simulink model "wk10_clsys"  (R2022b)
settings: Solver=VariableStepAuto  StartTime=0.0  StopTime=75  RelTol=1e-3
model workspace (MAT data in the model file):
  seed = 0
values from neighbouring files (symbols this model uses):
  Kd = 3    [wk10_clsys_script.m]
  Ki = 6    [wk10_clsys_script.m]
  Kp = 0.35    [wk10_clsys_script.m]
  s_eed = floor(rand(1)*100)    [wk10_clsys_script.m]
  sd_noise = 0.1    [wk10_clsys_script.m]
  tau_f = 70    [wk10_clsys_script.m]
settings Model: Creator=sd87  LastModifiedBy=agjri
settings ModelReferenceCC: EnableRefExpFcnMdlSchedulingChecks=on

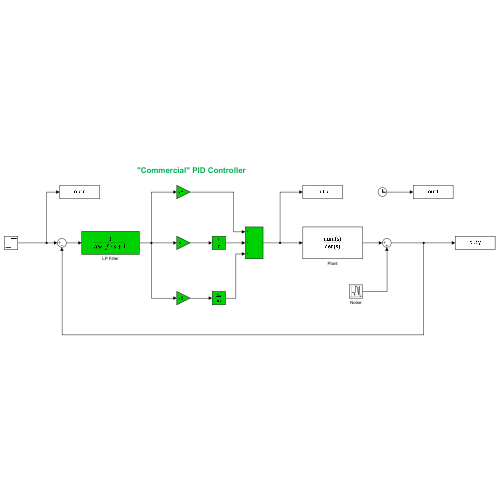
[thumbnail: Simulink's stored preview of the top-level diagram]
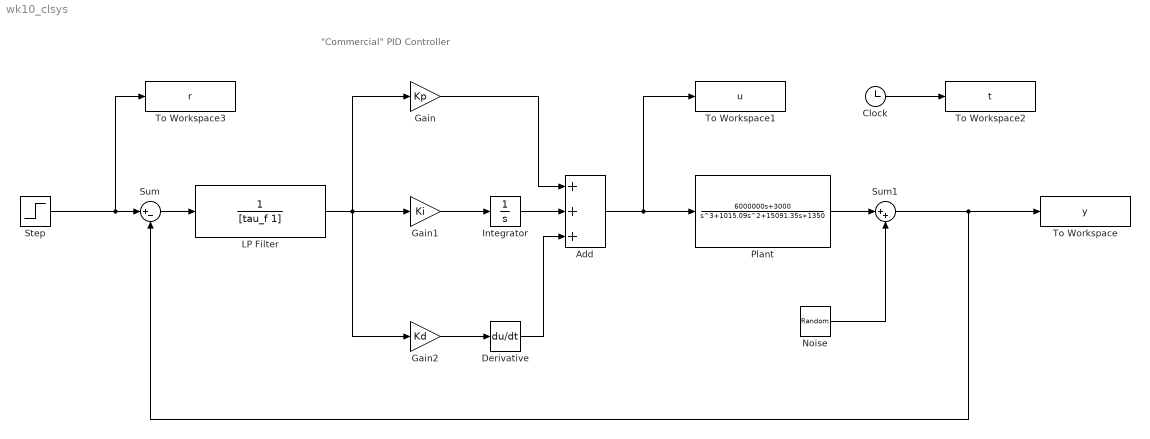
== system wk10_clsys ==
  note: "Commercial" PID Controller
  Add : Sum  Inputs=+++
  Clock : Clock
  Derivative : Derivative
  Gain : Gain  Gain=Kp
  Gain1 : Gain  Gain=Ki
  Gain2 : Gain  Gain=Kd
  Integrator : Integrator
  LP Filter : TransferFcn  Denominator=[tau_f 1]
  Noise : RandomNumber  Variance=sd_noise^2  Seed=s_eed  SampleTime=0.1
  Plant : TransferFcn  Numerator=[6000000 3000]  Denominator=[1 1015.09 15091.35 1350]
  Step : Step  SampleTime=0
  Sum : Sum  Inputs=|+-
  Sum1 : Sum  Inputs=|++
  To Workspace : ToWorkspace  VariableName=y  SampleTime=-1
  To Workspace1 : ToWorkspace  VariableName=u  SampleTime=-1
  To Workspace2 : ToWorkspace  VariableName=t  SampleTime=-1
  To Workspace3 : ToWorkspace  VariableName=r  SampleTime=-1
  wires:
  Clock/1 -> To Workspace2/1
  Step/1 -> To Workspace3/1, Sum/1
  Sum/1 -> LP Filter/1
  Add/1 -> To Workspace1/1, Plant/1
  Gain/1 -> Add/1
  Gain1/1 -> Integrator/1
  Integrator/1 -> Add/2
  Gain2/1 -> Derivative/1
  Derivative/1 -> Add/3
  LP Filter/1 -> Gain/1, Gain2/1, Gain1/1
  Plant/1 -> Sum1/1
  Sum1/1 -> To Workspace/1, Sum/2
  Noise/1 -> Sum1/2
